simulink model "experimental"  (R2016a)
settings: Solver=VariableStepAuto  StartTime=0.0  StopTime=200  FixedStep=0.001  RelTol=1e-3  SampleTimeConstraint=Specified
values from neighbouring files (symbols this model uses):
  a = 0.1329    [dynamics.m]    (also in setup.m; tire_test.m = 0.11372)
  b = 0.1221    [dynamics.m]    (also in setup.m; tire_test.m = 0.14328)
  C_alpha = 120000    [dynamics.m]    (also in setup.m; tire_test.m = 197)
  initial_states = [0 1 0]    [setup.m]
  Iz = 0.020899525    [dynamics.m]    (also in setup.m; tire_test.m = 0.025)
  L = 0.255    [dynamics.m]    (also in setup.m; tire_test.m = 0.257; veh_object2.m = obj_length)
  m = 2.622    [dynamics.m]    (also in setup.m; tire_test.m = 2.35)
  mu = 0.37    [dynamics.m]    (also in setup.m; tire_test.m = 1.31)
undefined symbols (not defined in the file): animation_update_interval, datetime, enable_CG_trace, enable_rearAxle_trace, plotAxisLimitMode, plotAxisLimits, save_anim_frames, vehicle_length, vehicle_width
libraries: vrlib x1, robotlib x1
settings Model: Creator=Cyrus  LastModifiedBy=Cyrus

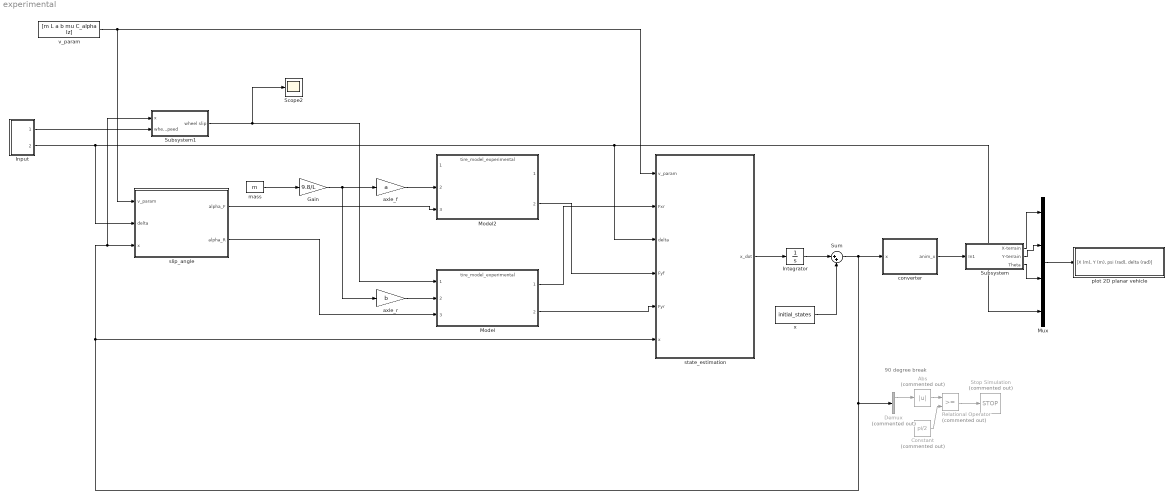
== system experimental ==
  note: 90 degree break
  Abs : Abs  Commented=on
  Constant : Constant  Commented=on  Value=pi/2
  Demux : Demux  Commented=on  Outputs=3
  Gain : Gain  Gain=9.8/L
  Input : Subsystem
  Integrator : Integrator
  Model : ModelReference  ModelNameDialog=tire_model_experimental.slx  SimulationMode=Normal  ModelReferenceVersion=1.2
  Model2 : ModelReference  ModelNameDialog=tire_model_experimental.slx  SimulationMode=Normal  ModelReferenceVersion=1.2
  Mux : Mux
  Relational Operator : RelationalOperator  Commented=on  OutDataTypeStr=boolean
  Scope2 : Scope
  Stop Simulation : Stop  Commented=on
  Subsystem : Subsystem
  Subsystem1 : Subsystem
  Sum : Sum  Inputs=|++
  axle_f : Gain  Gain=a
  axle_r : Gain  Gain=b
  converter : MATLAB Function  TreatAsAtomicUnit=on
  mass : Constant  Value=m
  plot 2D planar vehicle : Subsystem  mask(6DoF Animation){axisMode=plotAxisLimitMode, ax=plotAxisLimits, Ts=animation_update_interval, enable_CG_trace=enable_CG_trace, enable_rearAxle_trace=enable_rearAxle_trace, save_anim_frames=save_anim_frames, anim_frame_name_str=char(datetime('now','Format','yyyy-MM-dd_HH_mm_ss')), L=vehicle_length, W=vehicle_width}
      mask prompts: axisMode "Axis Mode (0->auto, 1->fixed, BOTH use Axes Limits below)"; ax "Axes limits [xmin xmax ymin ymax] (m):"; Ts "Time interval between updates (s):"; enable_CG_trace "Enable vehicle CG trace? (0/1)"; enable_rearAxle_trace "Enable rear axle trace? (0/1)"; save_anim_frames "Save animaton frames? (0/1)"; anim_frame_name_str "Animation sequence name (if save frames==1)"; L "Vehicle length (m)"; W "Vehicle width (m)"
      mask help:
      | Create a 2D animated view of a steering vehicle model with tires.
      |
      | Marc Compere
      | CompereM@saic.com
      | created : 22 August 2002
      | modified: 28 Dec 2015
      mask init:
      | Config.axisMode=axisMode;
      | Config.ax=ax;
      | Config.Ts=Ts;
      | Config.enable_CG_trace=enable_CG_trace;
      | Config.enable_rearAxle_trace=enable_rearAxle_trace;
      | Config.save_anim_frames=save_anim_frames;
      | Config.anim_frame_name_str=anim_frame_name_str;
      | Config.L=L;
      | Config.W=W;
      mask Help:
      | <p>This block generates a 3 dimensional display of a simulation trajectory, with the craft orientation displayed during flight</p>
      | 
      | <p>There are two inputs to this block, Position and Euler.  These inputs contain more than one signal as described below.</p>
      | 
      | <p><H4>Block Vector Input - Position</H4>
      | <ul>
      | <li>X Position</li>
      | <li>Y Position</li>
      | <li>Z Position</li>
      | </ul>
      | </p>
      | 
      | <p><H4>Block Vector Input - Euler</H4>
      |     <ul>
      |     <li>Roll Attitude</li>
      |     <li>Pitch Attitude</li>
      |     <li>Yaw Attitude</li>
      |    </ul>
      |    </p>
  slip_angle : MATLAB Function  TreatAsAtomicUnit=on
  state_estimation : MATLAB Function  TreatAsAtomicUnit=on
  v_param : Constant  Value=[m L a b mu C_alpha Iz]
  x : Constant  Value=initial_states
  wires:
  mass/1 -> Gain/1
  axle_f/1 -> Model2/2
  axle_r/1 -> Model/2
  Gain/1 -> axle_r/1, axle_f/1
  Sum/1 -> slip_angle/3(x), Subsystem1/1(x), state_estimation/6(x), Demux/1, converter/1(x)
  state_estimation/1(x_dot) -> Integrator/1
  Integrator/1 -> Sum/1
  x/1 -> Sum/2
  Subsystem/1(X-terrain) -> Mux/1
  Subsystem/2(Y-terrain) -> Mux/2
  Subsystem/3("Theta ") -> Mux/3
  Mux/1 -> plot 2D planar vehicle/1("[X (m), Y (m), psi (rad), delta (rad)]")
  v_param/1 -> state_estimation/1(v_param), slip_angle/1(v_param)
  Input/2(Steering) -> Mux/4, state_estimation/3(delta), slip_angle/2(delta)
  Demux/1 -> Abs/1
  Abs/1 -> Relational Operator/1
  Constant/1 -> Relational Operator/2
  Relational Operator/1 -> Stop Simulation/1
  Model2/2 -> state_estimation/4(Fyf)
  Model/2 -> state_estimation/5(Fyr)
  Model/1 -> state_estimation/2(Fxr)
  Subsystem1/1(wheel slip) -> Model/1, Scope2/1
  Input/1(Throttle) -> Subsystem1/2(wheel speed)
  slip_angle/2(alpha_R) -> Model/3
  slip_angle/1(alpha_F) -> Model2/3
  converter/1(anim_x) -> Subsystem/1(In1)

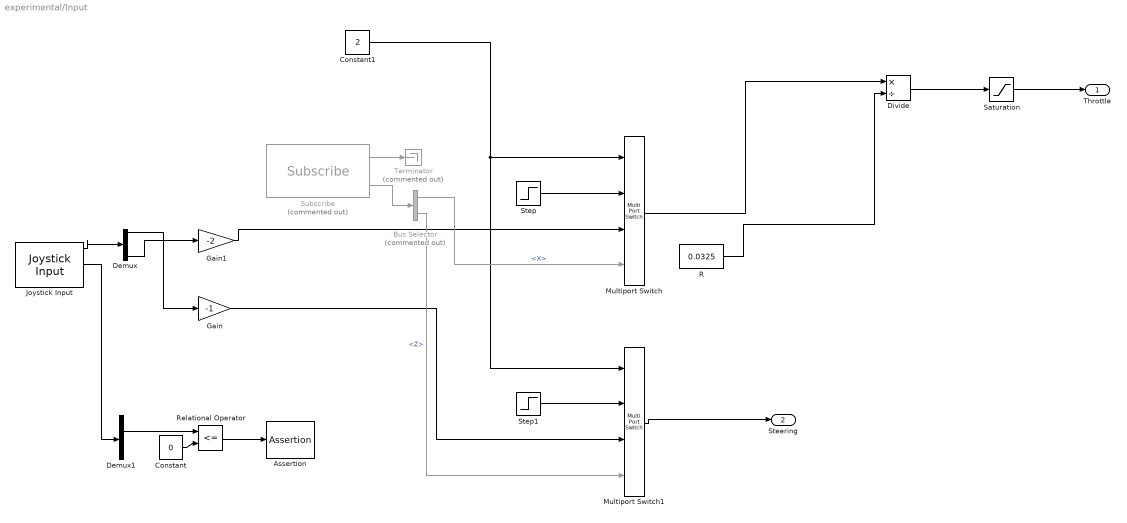
== system experimental/Input ==
  Assertion : Assertion  AssertionFailFcn=|  StopWhenAssertionFail=off
      | set_param(bdroot,'SimulationCommand','pause'),
      | disp(sprintf('\nSimulation paused.'))
  Bus Selector : BusSelector  Commented=on  OutputSignals=Linear.X,Angular.Z
  Constant : Constant  Value=0
  Constant1 : Constant  Value=2
  Demux : Demux
  Demux1 : Demux  Outputs=12
  Divide : Product  Inputs=*/
  Gain : Gain  Gain=-1  OutMin=[-1]  OutMax=[1]
  Gain1 : Gain  Gain=-2  OutMin=[0]  OutMax=[4]
  Joystick Input : vrlib/Joystick Input  joyid=1  adjustports=on  forcefeed=off
  Multiport Switch : MultiPortSwitch
  Multiport Switch1 : MultiPortSwitch
  R : Constant  Value=0.0325
  Relational Operator : RelationalOperator  Operator=<=  OutDataTypeStr=boolean
  Saturation : Saturate  UpperLimit=170  LowerLimit=0
  Step : Step  Time=3  Before=1.5  After=1.8  SampleTime=0
  Step1 : Step  After=0.73  SampleTime=0
  Subscribe : robotlib/Subscribe  Commented=on  SourceLibraryInfo=This block requires Robotics System Toolbox  topicSource=Select from ROS network  topic=/cmd_vel  messageType=geometry_msgs/Twist  sampleTime=-1  messageQueueLength=1
  Terminator : Terminator  Commented=on
  Throttle : Outport
  Steering : Outport  Port=2
  wires:
  Joystick Input/1 -> Demux/1
  Joystick Input/2 -> Demux1/1
  Demux1/5 -> Relational Operator/1
  Constant/1 -> Relational Operator/2
  Relational Operator/1 -> Assertion/1
  Multiport Switch1/1 -> Steering/1
  Constant1/1 -> Multiport Switch1/1, Multiport Switch/1
  Gain1/1 -> Multiport Switch/3
  Gain/1 -> Multiport Switch1/3
  Step/1 -> Multiport Switch/2
  Step1/1 -> Multiport Switch1/2
  Multiport Switch/1 -> Divide/1
  R/1 -> Divide/2
  Subscribe/1 -> Terminator/1
  Subscribe/2 -> Bus Selector/1
  Bus Selector/1 -> Multiport Switch/4  "<X>"
  Bus Selector/2 -> Multiport Switch1/4  "<Z>"
  Saturation/1 -> Throttle/1
  Divide/1 -> Saturation/1
  Demux/1 -> Gain/1
  Demux/4 -> Gain1/1

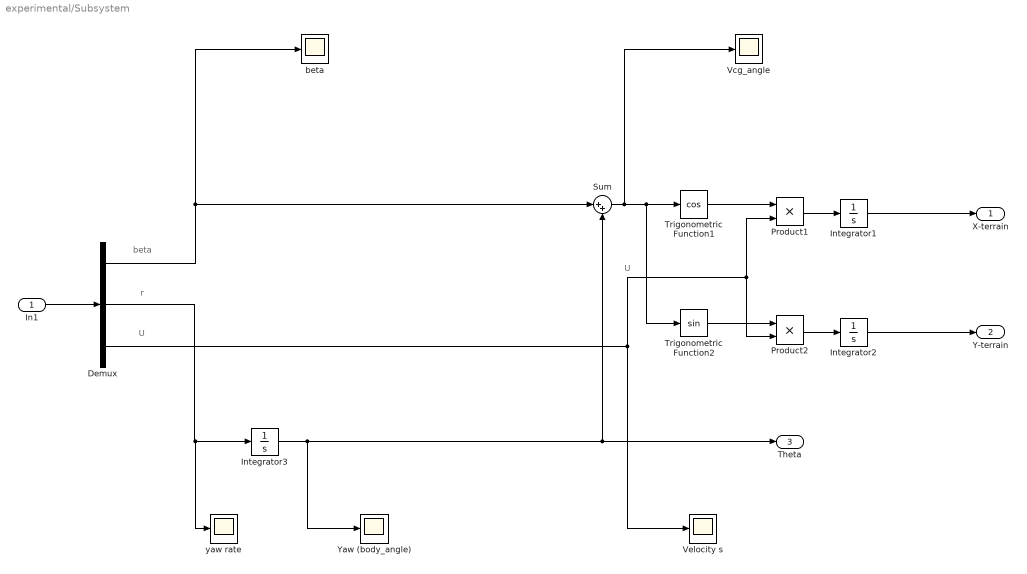
== system experimental/Subsystem ==
  note: r
  note: U
  note: U
  note: beta
  In1 : Inport
  Demux : Demux  Outputs=3
  Integrator1 : Integrator
  Integrator2 : Integrator
  Integrator3 : Integrator
  Product1 : Product
  Product2 : Product
  Sum : Sum  Inputs=|++
  Trigonometric Function1 : Trigonometry  Operator=cos
  Trigonometric Function2 : Trigonometry
  Vcg_angle : Scope
  Velocity s : Scope
  Yaw (body_angle) : Scope
  beta : Scope
  yaw rate : Scope
  X-terrain : Outport
  Y-terrain : Outport  Port=2
  "Theta " : Outport  Port=3
  wires:
  In1/1 -> Demux/1
  Demux/2 -> yaw rate/1, Integrator3/1
  Demux/1 -> Sum/1, beta/1
  Trigonometric Function1/1 -> Product1/1
  Trigonometric Function2/1 -> Product2/1
  Product1/1 -> Integrator1/1
  Product2/1 -> Integrator2/1
  Integrator1/1 -> X-terrain/1
  Integrator2/1 -> Y-terrain/1
  Integrator3/1 -> "Theta "/1, Sum/2, Yaw (body_angle)/1
  Sum/1 -> Vcg_angle/1, Trigonometric Function2/1, Trigonometric Function1/1
  Demux/3 -> Product1/2, Product2/2, Velocity s/1

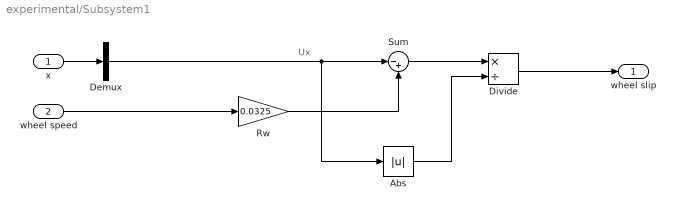
== system experimental/Subsystem1 ==
  note: Ux
  x : Inport
  wheel speed : Inport  Port=2
  Abs : Abs
  Demux : Demux  Outputs=3
  Divide : Product  Inputs=*/
  Rw : Gain  Gain=0.0325
  Sum : Sum  Inputs=|-+
  wheel slip : Outport
  wires:
  x/1 -> Demux/1
  wheel speed/1 -> Rw/1
  Sum/1 -> Divide/1
  Rw/1 -> Sum/2
  Abs/1 -> Divide/2
  Divide/1 -> wheel slip/1
  Demux/2 -> Abs/1, Sum/1

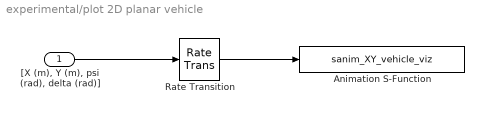
== system experimental/plot 2D planar vehicle ==
  "[X (m), Y (m), psi (rad), delta (rad)]" : Inport
  Animation S-Function : S-Function  FunctionName=sanim_XY_vehicle_viz  Parameters=Config  SFunctionDeploymentMode=off  EnableBusSupport=off
  Rate Transition : RateTransition  Integrity=off
  wires:
  "[X (m), Y (m), psi (rad), delta (rad)]"/1 -> Rate Transition/1
  Rate Transition/1 -> Animation S-Function/1

== matlab function experimental/state_estimation ==
  data: v_param input; Fxr input; delta input; Fyf input; Fyr input; x_dot output; x input
function x_dot  = veh_dyn(v_param,Fxr,delta,Fyf,Fyr,x)
%#codegen
m = v_param(1);
a = v_param(3);
b = v_param(4);
Iz = v_param(7);

r = x(1);
Ux = x(2);
Uy = x(3);

r_dot = (a*Fyf*cos(delta)-b*Fyr)/Iz;
Ux_dot = (Fxr-Fyf*sin(delta))/m+r*Uy;
Uy_dot = (Fyf*cos(delta)+Fyr)/m-r*Ux;

x_dot = [r_dot Ux_dot Uy_dot];

== matlab function experimental/slip_angle ==
  data: v_param input; delta input; x input; alpha_F output; alpha_R output
function [alpha_F, alpha_R] = slip_angle(v_param,delta,x)
%#codegen
a = v_param(3);
b = v_param(4);

r = x(1);
Ux = x(2);
Uy = x(3);


if Ux == 0 && Uy == 0   % vehicle is still no slip
    alpha_F = 0;
    alpha_R = 0;
elseif Ux == 0      % perfect side slip
    alpha_F = pi/2*sign(Uy)-delta;
    alpha_R = pi/2*sign(Uy);
elseif Ux < 0    % rare ken block situations
    alpha_F = (sign(Uy)*pi)-atan((Uy+a*r)/abs(Ux))-delta;
    alpha_R = (sign(Uy)*pi)-atan((Uy-b*r)/abs(Ux));
else                % normal situation
    alpha_F = atan((Uy+a*r)/abs(Ux))-delta;
    alpha_R = atan((Uy-b*r)/abs(Ux));
end

% safety that keep alpha in valid range
alpha_F = wrapToPi(alpha_F)
alpha_R = wrapToPi(alpha_R)


% if abs(Ux) <= 0.01
%     alpha_F = beta-delta;
%     alpha_R = beta;
% end
% if Uy+a*r > 100*Ux
%         alpha_F = pi/2-delta;
% elseif Uy+a*r < -100*Ux
%         alpha_F = -pi/2-delta;
% else
%         alpha_F = atan((Uy+a*r)/Ux)-delta;
% end
% 
% if Uy-b*r > 100*Ux
%     alpha_R = pi/2;
% elseif Uy-b*r < -100*Ux
%     alpha_R = -pi/2;
% else
%     alpha_R = atan((Uy-b*r)/Ux);
% end

== matlab function experimental/converter ==
  data: anim_x output; x input
function anim_x = converter(x)
r = x(1);
Ux = x(2);
Uy = x(3);

U = sqrt(Ux^2+Uy^2);
if Ux == 0 && Uy == 0
    beta = 0;
elseif Ux == 0
    beta = pi/2*sign(Uy);
elseif Ux < 0 && Uy == 0
    beta = pi;
elseif Ux < 0
    beta = sign(Uy)*pi-atan(Uy/abs(Ux));
else
    beta = atan(Uy/abs(Ux));
end
beta = wrapToPi(beta)

anim_x = [beta r U];
